simulink model "Servo_controller"  (R2021b)
settings: Solver=ode45  StartTime=0.0  StopTime=1  RelTol=1e-3
values from neighbouring files (symbols this model uses):
  KI = K(4)    [Project.m]
  Kp = K(1:3)    [Project.m]
  Ts = 0.02    [Project.m]
undefined symbols (not defined in the file or in its folder): Cz, G, H
settings Model: Creator=Amir  LastModifiedBy=Amir

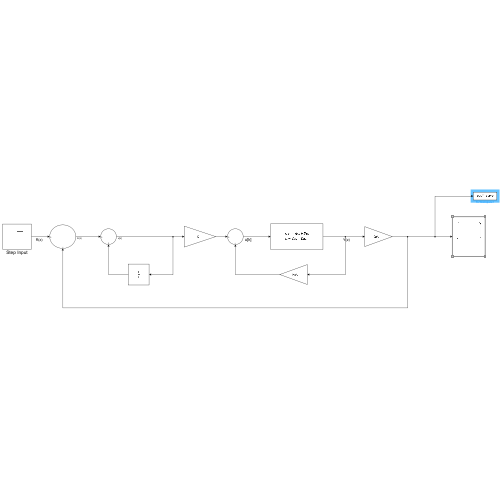
[thumbnail: Simulink's stored preview of the top-level diagram]
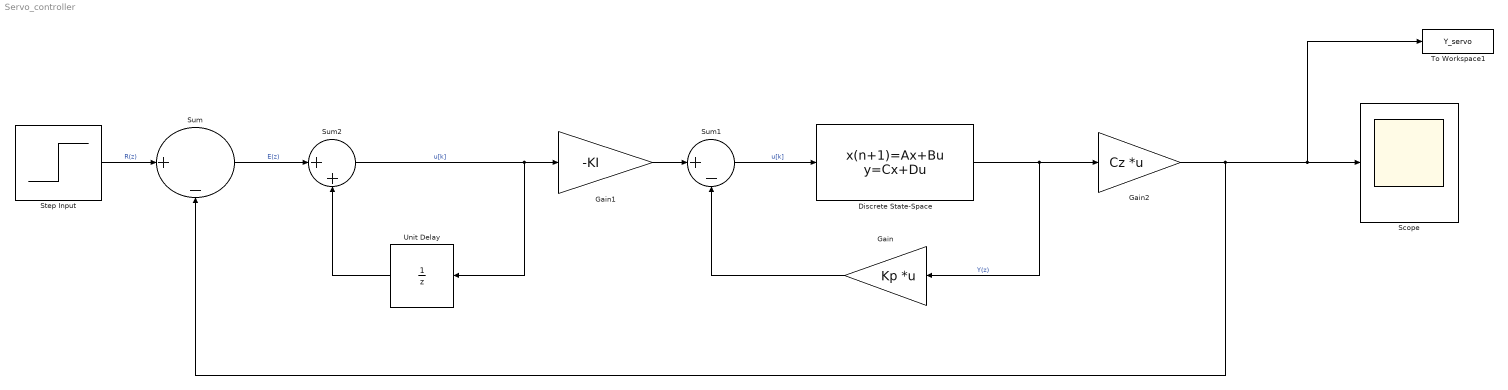
== system Servo_controller ==
  Discrete State-Space : DiscreteStateSpace  A=G  B=H  C=eye(3)  D=zeros(3,1)  SampleTime=Ts
  Gain : Gain  Gain=Kp  Multiplication=Matrix(K*u)
  Gain1 : Gain  Gain=-KI
  Gain2 : Gain  Gain=Cz  Multiplication=Matrix(K*u)
  Scope : Scope
  Step Input : Step  Time=0  After=0.01  SampleTime=0
  Sum : Sum  Inputs=|+-
  Sum1 : Sum  Inputs=|+-
  Sum2 : Sum  Inputs=|++
  To Workspace1 : ToWorkspace  VariableName=Y_servo  SaveFormat=Timeseries  SampleTime=-1
  Unit Delay : UnitDelay  SampleTime=-1  HasFrameUpgradeWarning=on
  wires:
  Discrete State-Space/1 -> Gain2/1, Gain/1  "Y(z)"
  Step Input/1 -> Sum/1  "R(z)"
  Sum1/1 -> Discrete State-Space/1  "u[k]"
  Gain/1 -> Sum1/2
  Gain1/1 -> Sum1/1
  Sum2/1 -> Unit Delay/1, Gain1/1  "u[k]"
  Sum/1 -> Sum2/1  "E(z)"
  Gain2/1 -> To Workspace1/1, Scope/1, Sum/2
  Unit Delay/1 -> Sum2/2
